simulink library "WECSim_Lib"  (R2014b)
settings: Solver=ode45  StartTime=0.0  StopTime=10.0  RelTol=1e-3
undefined symbols (not defined in the file): body, constraint, pto, simu, waves, X, Y, Z
libraries: nesl_utility x41, sm_lib x35
(part 2 of 2)

== system WECSim_Lib/PTOs/Translational PTO (Local Z) ==
  note: pto.loc
      | pto.c
      | pto.k
      | pto.name used in mask
  note: Constraints the motion to the desired DOF.
      | Applies PTO loads to the body based on PTO restoring and damping values.
      | Moves the connection points (B and F) from the free surface to the PTO location.
      | Calculates the PTO force and power.
      | Outputs forces, motions, and power.
  ForceAndPower : Subsystem
  Mux1 : Mux  Inputs=6
  PS-Simulink Converter{,1..3} (4 alike) : nesl_utility/PS-Simulink Converter  PhysicalDomain=network_engine_domain  SubClassName=ps_output  LeftPortType=input  RightPortType=output  PseudoPeriodic=off  Frequencies=[]  Unit=1  AffineConversion=off
  Rigid Transform : sm_lib/Frames and Transforms/Rigid Transform  TranslationMethod=Cartesian  TranslationLengthUnit=m  TranslationStandardAxis=+Z  TranslationStandardOffset=0  TranslationCartesianOffset=pto.loc  TranslationROffset=0  TranslationROffsetUnits=m  TranslationZOffset=0  TranslationZOffsetUnits=m  TranslationThetaOffset=0  TranslationThetaOffsetUnits=deg  RotationMethod=None  RotationAngleUnits=deg  RotationStandardAxis=+X  RotationAngle=90  RotationArbitraryAxis=[0 0 1]  FollAlignAxisA=+X  BaseAlignAxisA=+Y  FollAlignAxisB=+Y  BaseAlignAxisB=+Z  RotationMatrix=[1 0 0; 0 1 0; 0 0 1]  BlockFunction=simmechanics.library.frames_transforms.rigid_transform
  Rigid Transform1 : sm_lib/Frames and Transforms/Rigid Transform  TranslationMethod=Cartesian  TranslationLengthUnit=m  TranslationStandardAxis=+Z  TranslationStandardOffset=0  TranslationCartesianOffset=pto.loc  TranslationROffset=0  TranslationROffsetUnits=m  TranslationZOffset=0  TranslationZOffsetUnits=m  TranslationThetaOffset=0  TranslationThetaOffsetUnits=deg  RotationMethod=None  RotationAngleUnits=deg  RotationStandardAxis=+X  RotationAngle=90  RotationArbitraryAxis=[0 0 1]  FollAlignAxisA=+X  BaseAlignAxisA=+Y  FollAlignAxisB=+Y  BaseAlignAxisB=+Z  RotationMatrix=[1 0 0; 0 1 0; 0 0 1]  BlockFunction=simmechanics.library.frames_transforms.rigid_transform
  Translational PCC (Prismatic Joint) : sm_lib/Joints/Prismatic Joint  SenseConstraintForce=on  SenseConstraintForceX=off  SenseConstraintForceY=off  SenseConstraintForceZ=off  SenseConstraintTorque=on  SenseConstraintTorqueX=off  SenseConstraintTorqueY=off  SenseConstraintTorqueZ=off  SenseTotalForce=off  SenseTotalForceX=off  SenseTotalForceY=off  SenseTotalForceZ=off  SenseTotalTorque=off  SenseTotalTorqueX=off  SenseTotalTorqueY=off  SenseTotalTorqueZ=off  CompositeWrenchDir=BaseOnFollower  CompositeWrenchFrame=BaseFrame  EquilibriumPosition=0  EquilibriumPositionUnits=m  SpringStiffness=pto.k  SpringStiffnessUnits=N/m  DampingCoefficient=pto.c  DampingCoefficientUnits=N/(m/s)  TorqueActuationMode=NoTorque  MotionActuationMode=ComputedMotion  SensePosition=on  SenseVelocity=on  SenseAcceleration=off  SenseTorqueForce=off  PositionTargetValue=0  PositionTargetValueUnits=m  PositionTargetSpecify=off  PositionTargetPriority=High  VelocityTargetValue=0  VelocityTargetValueUnits=m/s  VelocityTargetSpecify=off  VelocityTargetPriority=High  BlockFunction=simmechanics.library.joints.prismatic_joint
  output : ToWorkspace  VariableName=PTO1_out  SaveFormat=Structure With Time  SampleTime=-1
  F : PMIOPort  Port=1  Side=Left
  B : PMIOPort  Port=2  Side=Right
  wires:
  PS-Simulink Converter1/1 -> Mux1/6, ForceAndPower/2(Vel)
  PS-Simulink Converter/1 -> Mux1/5, ForceAndPower/1(Pos)
  PS-Simulink Converter2/1 -> Mux1/3
  PS-Simulink Converter3/1 -> Mux1/4
  Mux1/1 -> output/1
  ForceAndPower/1(Force) -> Mux1/1
  ForceAndPower/2(Power) -> Mux1/2
  connections:
  Translational PCC (Prismatic Joint)/RConn3 -- PS-Simulink Converter1/LConn1
  Translational PCC (Prismatic Joint)/RConn2 -- PS-Simulink Converter/LConn1
  Translational PCC (Prismatic Joint)/RConn4 -- PS-Simulink Converter2/LConn1
  Translational PCC (Prismatic Joint)/RConn5 -- PS-Simulink Converter3/LConn1
  B/RConn1 -- Rigid Transform/LConn1
  Rigid Transform/RConn1 -- Translational PCC (Prismatic Joint)/LConn1
  Translational PCC (Prismatic Joint)/RConn1 -- Rigid Transform1/RConn1
  Rigid Transform1/LConn1 -- F/RConn1

== system WECSim_Lib/Body Elements/Rigid Body/Additional Linear Damping Force Calculation ==
  note: Calculates the additional linear damping force (if any)
      |
      | Additional Linear Damping Force = damping matrix (diagonal) * velocity vector = C * v
  Velocity : Inport
  Additional Linear Damping Matrix (diagonal) : Constant  Value=body.hydroForce.linearDamping
  Product1 : Product  Multiplication=Matrix(*)
  F_LinearDamping : Outport
  wires:
  Velocity/1 -> Product1/2  "v"
  Product1/1 -> F_LinearDamping/1  "F_LinearDamping"
  Additional Linear Damping Matrix (diagonal)/1 -> Product1/1  "C"

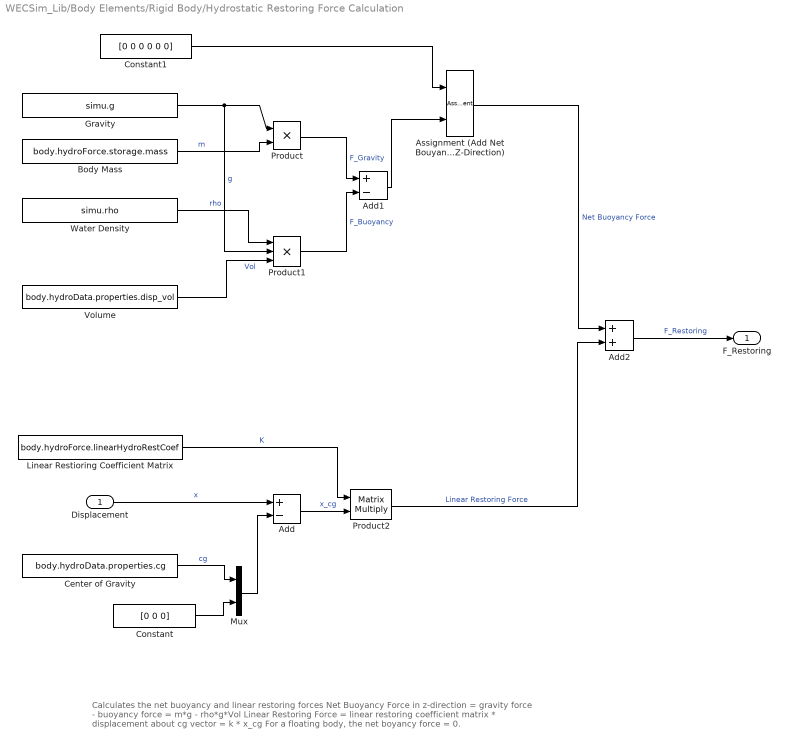
== system WECSim_Lib/Body Elements/Rigid Body/Hydrostatic Restoring Force Calculation ==
  note: Calculates the net buoyancy and linear restoring forces
      | 	Net Buoyancy Force in z-direction = gravity force - buoyancy force = m*g - rho*g*Vol
      | 	Linear Restoring Force = linear restoring coefficient matrix * displacement about cg vector = k * x_cg
      |
      | For a floating body, the net boyancy force = 0.
  Displacement : Inport
  Add : Sum  Inputs=+-
  Add1 : Sum  Inputs=+-
  Add2 : Sum
  Assignment (Add Net Bouyancy Force to Z-Direction) : Assignment  Indices=3
  Body Mass : Constant  Value=body.hydroForce.storage.mass
  Center of Gravity : Constant  Value=body.hydroData.properties.cg
  Constant : Constant  Value=[0 0 0]
  Constant1 : Constant  Value=[0 0 0 0 0 0]
  Gravity : Constant  Value=simu.g
  Linear Restioring Coefficient Matrix : Constant  Value=body.hydroForce.linearHydroRestCoef
  Mux : Mux  Inputs=2
  Product : Product
  Product1 : Product  Inputs=3
  Product2 : Product  Multiplication=Matrix(*)
  Volume : Constant  Value=body.hydroData.properties.disp_vol
  Water Density : Constant  Value=simu.rho
  F_Restoring : Outport
  wires:
  Add/1 -> Product2/2  "x_cg"
  Displacement/1 -> Add/1  "x"
  Mux/1 -> Add/2
  Center of Gravity/1 -> Mux/1  "cg"
  Constant/1 -> Mux/2
  Body Mass/1 -> Product/2  "m"
  Constant1/1 -> Assignment (Add Net Bouyancy Force to Z-Direction)/1
  Assignment (Add Net Bouyancy Force to Z-Direction)/1 -> Add2/1  "Net Buoyancy Force"
  Add2/1 -> F_Restoring/1  "F_Restoring"
  Volume/1 -> Product1/3  "Vol"
  Gravity/1 -> Product1/2, Product/1  "g"
  Water Density/1 -> Product1/1  "rho"
  Product/1 -> Add1/1  "F_Gravity"
  Product1/1 -> Add1/2  "F_Buoyancy"
  Add1/1 -> Assignment (Add Net Bouyancy Force to Z-Direction)/2
  Product2/1 -> Add2/2  "Linear Restoring Force"
  Linear Restioring Coefficient Matrix/1 -> Product2/1  "K"

== system WECSim_Lib/Body Elements/Rigid Body/Mooring Force Calculation (Map) ==
  note: Calculates the Mooring Force
      |
      | Mooring force = Kmooring matrix * displacement vector (relative to cg)
      | 	+ Cmooring matrix * velocity vector
      | 	- PreTension vector
      | F_Mooring = x_cg * Km  +  v * Cm  -  T
  Displacement : Inport
  Velocity : Inport  Port=2
  0 Disp for Rotation : Constant  Value=[0 0 0]
  Add : Sum  Inputs=+-
  Center of Gravity : Constant  Value=body.hydroData.properties.cg
  Center of Gravity2 : Constant  Value=body.mooring.c
  Mooring K Matrix : Constant  Value=body.mooring.k
  Mooring Pre-Tension : Constant  Value=body.mooring.preTension
  Mux : Mux  Inputs=2
  Product : Product  Multiplication=Matrix(*)
  Product1 : Product  Multiplication=Matrix(*)
  sum : Sum  Inputs=++-
  F_Mooring : Outport
  wires:
  Product/1 -> sum/1  "Km*x_cg"
  Product1/1 -> sum/2  "Cm*v"
  sum/1 -> F_Mooring/1  "F_Mooring"
  Mooring Pre-Tension/1 -> sum/3  "T"
  Add/1 -> Product/2  "x_cg"
  Mux/1 -> Add/2
  Displacement/1 -> Add/1  "x"
  Center of Gravity/1 -> Mux/1  "cg"
  Mooring K Matrix/1 -> Product/1  "Km"
  Velocity/1 -> Product1/2  "v"
  Center of Gravity2/1 -> Product1/1  "Cm"
  0 Disp for Rotation/1 -> Mux/2

== system WECSim_Lib/Body Elements/Rigid Body/Structure ==
  note: body.mass
      | body.momOfInertia
      | body.geometryFile (set through Rigid Body mask)
      | body.hydroData.properties.cg
      | body.initDisp.initAngularDispAxis
      | body.initDisp.initAngularDispAngle
      | body.initDisp.initLinDisp
  note: SimMechanics Model
      |
      | Body: Consists of body properties (inertia and vizualisation) defined at the CG, and a connection point at (0,0,0), the free surface.
      |
      | Forces::  Total forces calculated by WEC-Sim are applied at the Body CG. Other forces (constraints and PTOs) can be applied outside of this block, though the connection point.
      |
      | Motion Sensor: Measures the displacement, velocity, and acceleration of the Body CG relative to the world frame.
  Total Force : Inport
  Body Properties : sm_lib/Body Elements/Solid  InertiaType=Custom  Mass=body.mass  MassUnits=kg  CenterOfMass=[0 0 0]  CenterOfMassUnits=m  MomentsOfInertia=body.momOfInertia  MomentsOfInertiaUnits=kg*m^2  ProductsOfInertia=[0 0 0]  ProductsOfInertiaUnits=kg*m^2  DensityBased=on  Density=1000  DensityUnits=kg/(m^3)  GraphicType=FromGeometry  MarkerShape=Sphere  MarkerSize=10  MarkerSizeUnits=m  GraphicVisPropType=SimpleVisualProperties  GraphicDiffuseColor=[1 1 0]  GraphicSpecularColor=[0.5 0.5 0.5 1.0]  GraphicAmbientColor=[0.15 0.15 0.15 1.0]  GraphicEmissiveColor=[0.0 0.0 0.0 1.0]  GraphicShininess=75  GraphicOpacity=1  GeometryShape=FromFile  RectangleSize=[1 1]  RectangleSizeUnits=m  BrickDimensions=[1 1 1]  BrickDimensionUnits=m  CylinderRadius=1  CylinderRadiusUnits=m  CylinderLength=1  CylinderLengthUnits=m  SphereRadius=1  SphereRadiusUnits=m  EllipsoidRadii=[1 1 1]  EllipsoidRadiiUnits=m  ExtrusionCrossSection=[1 1; -1 1; -1 -1; 1 -1]  ExtrusionCrossSectionUnits=m  ExtrusionLength=1  ExtrusionLengthUnits=m  PolygonNumSides=3  PolygonOuterRadius=1  PolygonOuterRadiusUnits=m  ExtGeomFileType=STL  ExtGeomFileName=geometry/flap.stl  ExtGeomFileUnits=m  RevolutionCrossSection=[1 1; 1 -1; 2 -1; 2 1]  RevolutionCrossSectionUnits=m  RevolutionExtent=Full  RevolutionAngle=180  RevolutionAngleUnits=deg  BlockFunction=simmechanics.library.body_elements.solid
  External Force and Torque : sm_lib/Forces and Torques/External Force and Torque  ForceResolutionFrame=AttachedFrame  EnableForceX=off  EnableForceY=off  EnableForceZ=off  EnableForce=on  TorqueResolutionFrame=AttachedFrame  EnableTorqueX=off  EnableTorqueY=off  EnableTorqueZ=off  EnableTorque=on  BlockFunction=simmechanics.library.forces_torques.external_force_torque
  Motion Sensor : Subsystem
  Rigid Transform (Setup CG) : sm_lib/Frames and Transforms/Rigid Transform  TranslationMethod=Cartesian  TranslationLengthUnit=m  TranslationStandardAxis=+Z  TranslationStandardOffset=0  TranslationCartesianOffset=body.hydroData.properties.cg  TranslationROffset=0  TranslationROffsetUnits=m  TranslationZOffset=0  TranslationZOffsetUnits=m  TranslationThetaOffset=0  TranslationThetaOffsetUnits=deg  RotationMethod=None  RotationAngleUnits=rad  RotationStandardAxis=+Y  RotationAngle=0.05  RotationArbitraryAxis=[0.57735026918962584 0.57735026918962584 0.57735026918962584]  FollAlignAxisA=+X  BaseAlignAxisA=+Y  FollAlignAxisB=+Y  BaseAlignAxisB=+Z  RotationMatrix=[1 0 0; 0 1 0; 0 0 1]  BlockFunction=simmechanics.library.frames_transforms.rigid_transform
  Rigid Transform (Setup Initial Disp) : sm_lib/Frames and Transforms/Rigid Transform  TranslationMethod=Cartesian  TranslationLengthUnit=m  TranslationStandardAxis=+Z  TranslationStandardOffset=0  TranslationCartesianOffset=body.initDisp.initLinDisp  TranslationROffset=0  TranslationROffsetUnits=m  TranslationZOffset=0  TranslationZOffsetUnits=m  TranslationThetaOffset=0  TranslationThetaOffsetUnits=deg  RotationMethod=ArbitraryAxis  RotationAngleUnits=rad  RotationStandardAxis=+Y  RotationAngle=body.initDisp.initAngularDispAngle  RotationArbitraryAxis=body.initDisp.initAngularDispAxis  FollAlignAxisA=+X  BaseAlignAxisA=+Y  FollAlignAxisB=+Y  BaseAlignAxisB=+Z  RotationMatrix=[1 0 0; 0 1 0; 0 0 1]  BlockFunction=simmechanics.library.frames_transforms.rigid_transform
  Selector : Selector  InputPortWidth=6  Indices=[1:3]
  Selector1 : Selector  InputPortWidth=6  Indices=[4:6]
  Simulink-PS Converter1 : nesl_utility/Simulink-PS Converter  PhysicalDomain=network_engine_domain  SubClassName=ps_input  LeftPortType=input  RightPortType=output  PseudoPeriodic=off  Frequencies=[]  NoiseDistribution=none  NoiseParameters=[]  Unit=1  AffineConversion=off  InputFiltering=off  SimscapeFilterOrder=1  InputFilterTimeConstant=0.001  UdotUserProvided=1
  Simulink-PS Converter2 : nesl_utility/Simulink-PS Converter  PhysicalDomain=network_engine_domain  SubClassName=ps_input  LeftPortType=input  RightPortType=output  PseudoPeriodic=off  Frequencies=[]  NoiseDistribution=none  NoiseParameters=[]  Unit=1  AffineConversion=off  InputFiltering=off  SimscapeFilterOrder=1  InputFilterTimeConstant=0.001  UdotUserProvided=1
  World Frame : sm_lib/Frames and Transforms/World Frame  BlockFunction=simmechanics.library.frames_transforms.world_frame
  Conn Free Surface : PMIOPort  Port=1  Side=Right
  Response : Outport
  wires:
  Total Force/1 -> Selector1/1, Selector/1
  Selector/1 -> Simulink-PS Converter1/1
  Selector1/1 -> Simulink-PS Converter2/1
  Motion Sensor/1(Response) -> Response/1
  connections:
  External Force and Torque/LConn1 -- Simulink-PS Converter1/RConn1
  External Force and Torque/LConn2 -- Simulink-PS Converter2/RConn1
  Rigid Transform (Setup Initial Disp)/RConn1 -- Body Properties/RConn1 -- External Force and Torque/RConn1 -- Motion Sensor/RConn1
  Conn Free Surface/RConn1 -- Rigid Transform (Setup CG)/LConn1
  Rigid Transform (Setup Initial Disp)/LConn1 -- Rigid Transform (Setup CG)/RConn1
  World Frame/RConn1 -- Motion Sensor/LConn1

== system WECSim_Lib/Body Elements/Rigid Body/Viscous Damping Force Calculation ==
  note: Calculates Viscous Drag (Quadratic) Force
      |
      | Viscous Drag Force = 1/2 * drag coefficient * water density * characteristic area * velocity squared (signed) = 0.5 * cd * rho *A * v * |v|
  Velocity : Inport
  Abs : Abs
  Product : Product
  Product1 : Product  Multiplication=Matrix(*)
  "Viscous Damping Matrix (diagonal) " : Constant  Value=body.hydroForce.visDrag
  F_Viscous : Outport
  wires:
  Velocity/1 -> Product/1, Abs/1
  Abs/1 -> Product/2
  Product1/1 -> F_Viscous/1  "F_Viscous"
  "Viscous Damping Matrix (diagonal) "/1 -> Product1/1  "0.5 * cd * rho *A"
  Product/1 -> Product1/2  "v * |v|"

== system WECSim_Lib/Body Elements/Rigid Body/Wave Diffraction and Excitation Force Calculation ==
  note: Calculates the excitation force, F_Excitation, given by
      | F_Excitation = R * F_wave.
      |
      | There are two cases for Calculating the Ramp function, R:
      |    1. simulation Time is less than Ramp Time: Apply ramp function
      |    2. Simulation time is larger than Ramp Time: Do not apply ramp function (R=1)
      |
      | Similarly there are two cases for the wave force, F_wave: Regular and Irregular waves.
      |
      | Notes:
      | Output dimension set to '6' in output port to eliminate singleton dimension.
  Time : Inport
  If : If  IfExpression=u1 < 20
  If1 : If  NumInputs=2  IfExpression=u1 < u2
  Iregular Wave Excitation Force : Subsystem  TreatAsAtomicUnit=on
  Merge : Merge
  Merge1 : Merge
  No Ramp Function : Subsystem  TreatAsAtomicUnit=on
  Product : Product
  Ramp Function : Subsystem  TreatAsAtomicUnit=on
  Ramp Function Time : Constant  Value=simu.rampT
  Regular Wave Excitation Force : Subsystem  TreatAsAtomicUnit=on
  Wave Type : Constant  Value=waves.typeNum
  F_Excitation : Outport  PortDimensions=6
  wires:
  No Ramp Function/1(R) -> Merge1/2
  Ramp Function/1(R) -> Merge1/1
  If1/1 -> Ramp Function/Action
  If1/2 -> No Ramp Function/Action
  Ramp Function Time/1 -> If1/2
  Iregular Wave Excitation Force/1(F_wave) -> Merge/2
  Regular Wave Excitation Force/1(F_wave) -> Merge/1
  If/2 -> Iregular Wave Excitation Force/Action
  If/1 -> Regular Wave Excitation Force/Action
  Wave Type/1 -> If/1
  Merge/1 -> Product/2  "F_wave"
  Merge1/1 -> Product/1  "R"
  Product/1 -> F_Excitation/1  "F_Excitation"
  Time/1 -> Ramp Function/1(Time), If1/1, Iregular Wave Excitation Force/1(Time), Regular Wave Excitation Force/1(Time)

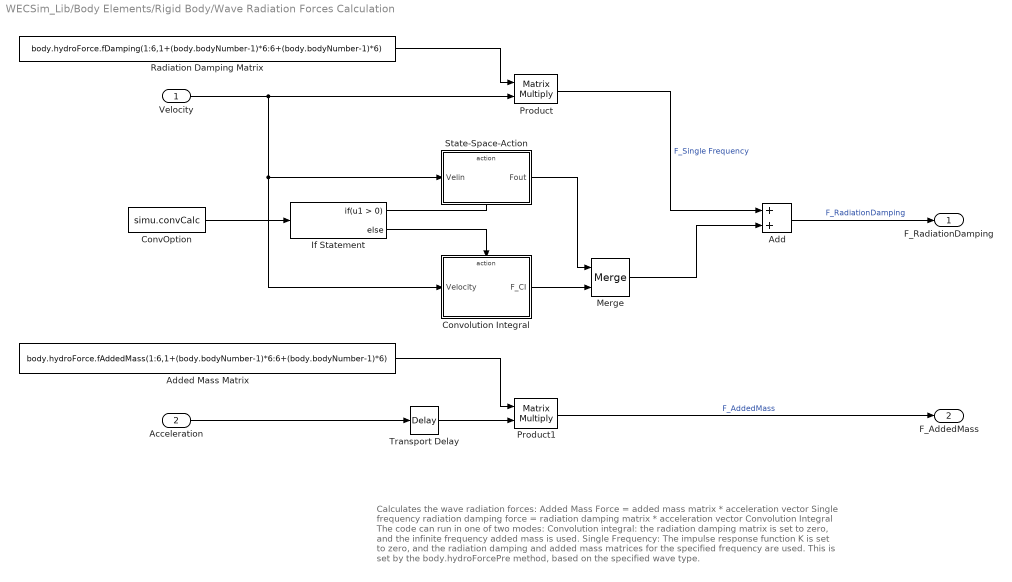
== system WECSim_Lib/Body Elements/Rigid Body/Wave Radiation Forces Calculation ==
  note: Calculates the wave radiation forces:
      | 	Added Mass Force = added mass matrix * acceleration vector
      | 	Single frequency radiation damping force = radiation damping matrix * acceleration vector
      | 	Convolution Integral
      |
      | The code can run in one of two modes:
      | 	Convolution integral: the radiation damping matrix is set to zero, and the infinite frequency added mass is used.
      | 	Single Frequency: The impulse response function K is set to zero, and the radiation damping and added mass matrices for the specified frequency are used.
      |
      | This is set by the body.hydroForcePre method, based on the specified wave type.
  Velocity : Inport
  Acceleration : Inport  Port=2
  Add : Sum
  Added Mass Matrix : Constant  Value=body.hydroForce.fAddedMass(1:6,1+(body.bodyNumber-1)*6:6+(body.bodyNumber-1)*6)
  ConvOption : Constant  Value=simu.convCalc
  Convolution Integral : Subsystem
  If Statement : If
  Merge : Merge
  Product : Product  Multiplication=Matrix(*)
  Product1 : Product  Multiplication=Matrix(*)
  Radiation Damping Matrix : Constant  Value=body.hydroForce.fDamping(1:6,1+(body.bodyNumber-1)*6:6+(body.bodyNumber-1)*6)
  State-Space-Action : Subsystem  TreatAsAtomicUnit=on
  Transport Delay : TransportDelay  DelayTime=10e-8
  F_RadiationDamping : Outport
  F_AddedMass : Outport  Port=2
  wires:
  Acceleration/1 -> Transport Delay/1
  Transport Delay/1 -> Product1/2
  Add/1 -> F_RadiationDamping/1  "F_RadiationDamping"
  Velocity/1 -> Convolution Integral/1(Velocity), State-Space-Action/1(Velin), Product/2
  Product/1 -> Add/1  "F_Single Frequency"
  Product1/1 -> F_AddedMass/1  "F_AddedMass"
  Radiation Damping Matrix/1 -> Product/1
  Added Mass Matrix/1 -> Product1/1
  If Statement/2 -> Convolution Integral/Action
  If Statement/1 -> State-Space-Action/Action
  State-Space-Action/1(Fout) -> Merge/1
  Convolution Integral/1(F_CI) -> Merge/2
  ConvOption/1 -> If Statement/1
  Merge/1 -> Add/2

== system WECSim_Lib/PTOs/Rotational PTO (Local RY)/ForceAndPower ==
  note: Calculate PTO force and power.
      |
      | F_pto  = k*x + c*v,
      | where F_pto is the force the PTO applies to the body (at the PTO location), x and v are the joint position and velocity.
      |
      | The power extracted is
      | P = c * v^2
  Pos : Inport
  Vel : Inport  Port=2
  Add : Sum
  Math Function : Math  Operator=square  SaturateOnIntegerOverflow=on
  PCC Damping Coefficient : Constant  Value=pto.c
  PCC Stiffness Coefficient : Constant  Value=pto.k
  Product : Product  Inputs=**
  Product1 : Product  Inputs=**
  Product2 : Product  Inputs=**
  Force/Torque : Outport
  Power : Outport  Port=2
  wires:
  PCC Damping Coefficient/1 -> Product2/1, Product1/1
  Product2/1 -> Power/1
  Vel/1 -> Math Function/1, Product1/2
  PCC Stiffness Coefficient/1 -> Product/2
  Pos/1 -> Product/1
  Add/1 -> Force/Torque/1
  Math Function/1 -> Product2/2
  Product/1 -> Add/1
  Product1/1 -> Add/2

== system WECSim_Lib/PTOs/Translational PTO (Local X)/ForceAndPower ==
  note: Calculate PTO force and power.
      |
      | F_pto  = k*x + c*v,
      | where F_pto is the force the PTO applies to the body (at the PTO location), x and v are the joint position and velocity.
      |
      | The power extracted is
      | P = c * v^2
  Pos : Inport
  Vel : Inport  Port=2
  Add : Sum
  Math Function : Math  Operator=square  SaturateOnIntegerOverflow=on
  PCC Damping Coefficient : Constant  Value=pto.c
  PCC Stiffness Coefficient : Constant  Value=pto.k
  Product : Product  Inputs=**
  Product1 : Product  Inputs=**
  Product2 : Product  Inputs=**
  Force : Outport
  Power : Outport  Port=2
  wires:
  PCC Damping Coefficient/1 -> Product1/1, Product2/1
  Product2/1 -> Power/1
  Vel/1 -> Product1/2, Math Function/1
  PCC Stiffness Coefficient/1 -> Product/2
  Pos/1 -> Product/1
  Add/1 -> Force/1
  Math Function/1 -> Product2/2
  Product/1 -> Add/1
  Product1/1 -> Add/2

== system WECSim_Lib/PTOs/Translational PTO (Local Z)/ForceAndPower ==
  note: Calculate PTO force and power.
      |
      | F_pto  = k*x + c*v,
      | where F_pto is the force the PTO applies to the body (at the PTO location), x and v are the joint position and velocity.
      |
      | The power extracted is
      | P = c * v^2
  Pos : Inport
  Vel : Inport  Port=2
  Add : Sum
  Math Function : Math  Operator=square  SaturateOnIntegerOverflow=on
  PCC Damping Coefficient : Constant  Value=pto.c
  PCC Stiffness Coefficient : Constant  Value=pto.k
  Product : Product  Inputs=**
  Product1 : Product  Inputs=**
  Product2 : Product  Inputs=**
  Force : Outport
  Power : Outport  Port=2
  wires:
  PCC Damping Coefficient/1 -> Product2/1, Product1/1
  Product2/1 -> Power/1
  Vel/1 -> Math Function/1, Product1/2
  PCC Stiffness Coefficient/1 -> Product/2
  Pos/1 -> Product/1
  Add/1 -> Force/1
  Math Function/1 -> Product2/2
  Product/1 -> Add/1
  Product1/1 -> Add/2

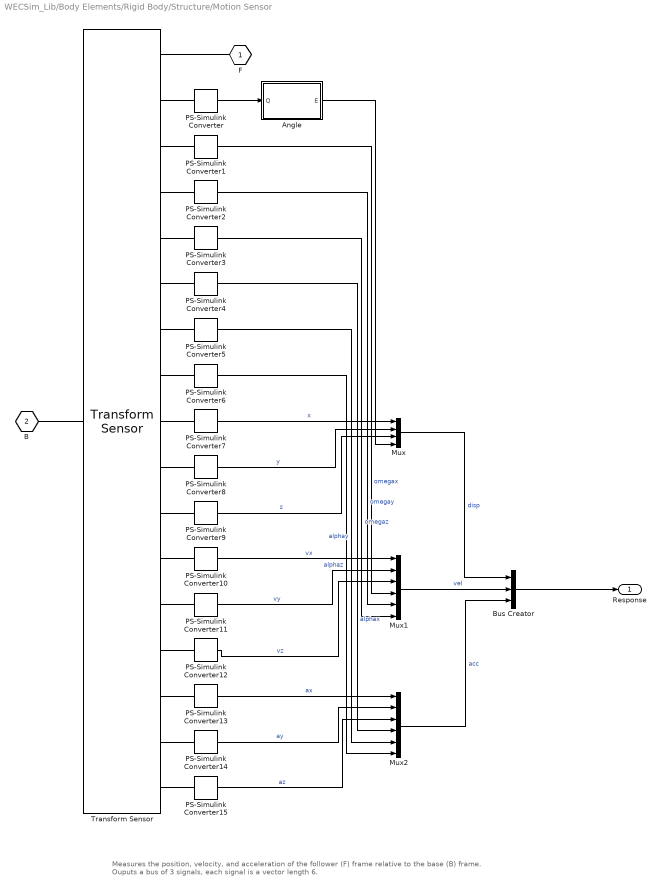
== system WECSim_Lib/Body Elements/Rigid Body/Structure/Motion Sensor ==
  note: Measures the position, velocity, and acceleration of the follower (F) frame relative to the base (B) frame.
      | Ouputs a bus of 3 signals, each signal is a vector length 6.
  Angle : MATLAB Function  TreatAsAtomicUnit=on
  Bus Creator : BusCreator  Inputs=3
  Mux : Mux
  Mux1 : Mux  Inputs=6
  Mux2 : Mux  Inputs=6
  PS-Simulink Converter{,1..15} (16 alike) : nesl_utility/PS-Simulink Converter  PhysicalDomain=network_engine_domain  SubClassName=ps_output  LeftPortType=input  RightPortType=output  PseudoPeriodic=off  Frequencies=[]  Unit=1  AffineConversion=off
  Transform Sensor : sm_lib/Frames and Transforms/Transform Sensor  MeasurementFrame=World  SenseAngle=off  SenseAxis=off  SenseAngle1=off  SenseAngle2=off  SenseAngle3=off  SenseQ=on  SenseR=off  SenseOmegaX=on  SenseOmegaY=on  SenseOmegaZ=on  SenseOmega1=off  SenseOmega2=off  SenseOmega3=off  SenseQDot=off  SenseRDot=off  SenseAlphaX=on  SenseAlphaY=on  SenseAlphaZ=on  SenseAlpha1=off  SenseAlpha2=off  SenseAlpha3=off  SenseQDDot=off  SenseRDDot=off  SenseX=on  SenseY=on  SenseZ=on  SenseRad=off  SenseAzim=off  SenseDist=off  SenseInc=off  SenseXDot=on  SenseYDot=on  SenseZDot=on  SenseRadDot=off  SenseAzimDot=off  SenseDistDot=off  SenseIncDot=off  SenseXDDot=on  SenseYDDot=on  SenseZDDot=on  SenseRadDDot=off  SenseAzimDDot=off  SenseDistDDot=off  SenseIncDDot=off  BlockFunction=simmechanics.library.frames_transforms.transform_sensor
  F : PMIOPort  Port=1  Side=Right
  B : PMIOPort  Port=2  Side=Left
  Response : Outport
  wires:
  PS-Simulink Converter/1 -> Angle/1(Q)
  PS-Simulink Converter4/1 -> Mux2/4  "alphax"
  PS-Simulink Converter10/1 -> Mux1/1  "vx"
  PS-Simulink Converter12/1 -> Mux1/3  "vz"
  PS-Simulink Converter13/1 -> Mux2/1  "ax"
  PS-Simulink Converter14/1 -> Mux2/2  "ay"
  Mux/1 -> Bus Creator/1  "disp"
  Mux1/1 -> Bus Creator/2  "vel"
  Mux2/1 -> Bus Creator/3  "acc"
  Angle/1(E) -> Mux/4
  PS-Simulink Converter7/1 -> Mux/1  "x"
  PS-Simulink Converter8/1 -> Mux/2  "y"
  PS-Simulink Converter9/1 -> Mux/3  "z"
  PS-Simulink Converter5/1 -> Mux2/5  "alphay"
  PS-Simulink Converter6/1 -> Mux2/6  "alphaz"
  PS-Simulink Converter1/1 -> Mux1/4  "omegax"
  PS-Simulink Converter2/1 -> Mux1/5  "omegay"
  PS-Simulink Converter11/1 -> Mux1/2  "vy"
  PS-Simulink Converter3/1 -> Mux1/6  "omegaz"
  PS-Simulink Converter15/1 -> Mux2/3  "az"
  Bus Creator/1 -> Response/1
  connections:
  Transform Sensor/RConn1 -- F/RConn1
  B/RConn1 -- Transform Sensor/LConn1
  Transform Sensor/RConn2 -- PS-Simulink Converter/LConn1
  PS-Simulink Converter15/LConn1 -- Transform Sensor/RConn17
  PS-Simulink Converter14/LConn1 -- Transform Sensor/RConn16
  PS-Simulink Converter13/LConn1 -- Transform Sensor/RConn15
  PS-Simulink Converter12/LConn1 -- Transform Sensor/RConn14
  PS-Simulink Converter11/LConn1 -- Transform Sensor/RConn13
  PS-Simulink Converter10/LConn1 -- Transform Sensor/RConn12
  PS-Simulink Converter9/LConn1 -- Transform Sensor/RConn11
  PS-Simulink Converter8/LConn1 -- Transform Sensor/RConn10
  PS-Simulink Converter7/LConn1 -- Transform Sensor/RConn9
  PS-Simulink Converter4/LConn1 -- Transform Sensor/RConn6
  PS-Simulink Converter5/LConn1 -- Transform Sensor/RConn7
  PS-Simulink Converter6/LConn1 -- Transform Sensor/RConn8
  PS-Simulink Converter1/LConn1 -- Transform Sensor/RConn3
  PS-Simulink Converter2/LConn1 -- Transform Sensor/RConn4
  PS-Simulink Converter3/LConn1 -- Transform Sensor/RConn5

== system WECSim_Lib/Body Elements/Rigid Body/Wave Diffraction and Excitation Force Calculation/Iregular Wave Excitation Force ==
  note: Calculates the wave force, F_wave, for the case of Irregular Waves.
      |
      | F_wave = sum( F_wave(i))
      |
      | where i = each frequency bin.
  Time : Inport
  Action Port : ActionPort
  For Each Subsystem : Subsystem  TreatAsAtomicUnit=on
  Imaginary Part of Wave Excitation : Constant  Value=body.hydroForce.fExt.im  VectorParams1D=off
  Random Phase : Constant  Value=waves.phaseRand  VectorParams1D=off
  Real Part of Wave Excitation : Constant  Value=body.hydroForce.fExt.re  VectorParams1D=off
  Sum of Elements : Sum  Inputs=+  CollapseMode=Specified dimension
  Wave Frequency : Constant  Value=waves.w  VectorParams1D=off
  Wave Spectrum : Constant  Value=waves.A  VectorParams1D=off
  F_wave : Outport
  wires:
  Random Phase/1 -> For Each Subsystem/5(Random Phase)
  Sum of Elements/1 -> F_wave/1
  For Each Subsystem/1(F_wave(i)) -> Sum of Elements/1
  Wave Frequency/1 -> For Each Subsystem/2(Wave Frequency)
  Imaginary Part of Wave Excitation/1 -> For Each Subsystem/4(Imaginary Part of Wave Excitation)
  Real Part of Wave Excitation/1 -> For Each Subsystem/3(Real Part of Wave Excitation)
  Wave Spectrum/1 -> For Each Subsystem/1(Wave Spectrum)
  Time/1 -> For Each Subsystem/6(Time)

== system WECSim_Lib/Body Elements/Rigid Body/Wave Diffraction and Excitation Force Calculation/No Ramp Function ==
  note: No ramp function applied.
      | R = 1
      |
      | Note:
      | Output port initial value also set to 1,
  Action Port : ActionPort
  Constant : Constant
  R : Outport  InitialOutput=1
  wires:
  Constant/1 -> R/1

== system WECSim_Lib/Body Elements/Rigid Body/Wave Diffraction and Excitation Force Calculation/Ramp Function ==
  note: Calculates the ramp function, R, given by
      |
      | R = (1 / 2)  * (1 + sin( (pi / t_ramp) * t  +  ((3 / 2) * pi) ) ).
  Time : Inport
  Action Port : ActionPort
  Add : Sum
  Add1 : Sum
  Constant : Constant  Value=1/2
  Constant1 : Constant
  Constant2 : Constant  Value=3*pi/2
  Constant3 : Constant  Value=pi
  Divide : Product  Inputs=*/
  Product : Product
  Product1 : Product
  Ramp Time : Constant  Value=simu.rampT
  Sine Wave Function : Sin  TimeSource=Use external signal  SampleTime=0
  R : Outport
  wires:
  Add/1 -> Product/1
  Sine Wave Function/1 -> Add/2
  Constant1/1 -> Add/1
  Constant/1 -> Product/2
  Product/1 -> R/1
  Time/1 -> Product1/1  "t"
  Ramp Time/1 -> Divide/2  "t_ramp"
  Constant2/1 -> Add1/2  "phase"
  Add1/1 -> Sine Wave Function/1
  Product1/1 -> Add1/1
  Constant3/1 -> Divide/1
  Divide/1 -> Product1/2  "frequency"

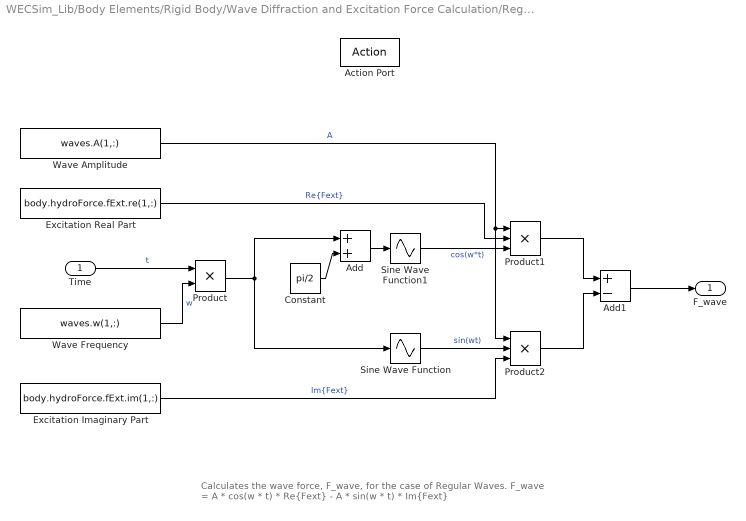
== system WECSim_Lib/Body Elements/Rigid Body/Wave Diffraction and Excitation Force Calculation/Regular Wave Excitation Force ==
  note: Calculates the wave force, F_wave, for the case of Regular Waves.
      |
      | F_wave =   A * cos(w * t) * Re{Fext}
      |                -  A * sin(w * t) * Im{Fext}
  Time : Inport
  Action Port : ActionPort
  Add : Sum
  Add1 : Sum  Inputs=+-
  Constant : Constant  Value=pi/2
  Excitation Imaginary Part : Constant  Value=body.hydroForce.fExt.im(1,:)  VectorParams1D=off
  Excitation Real Part : Constant  Value=body.hydroForce.fExt.re(1,:)  VectorParams1D=off
  Product : Product
  Product1 : Product  Inputs=3
  Product2 : Product  Inputs=3
  Sine Wave Function : Sin  TimeSource=Use external signal  SampleTime=0
  Sine Wave Function1 : Sin  TimeSource=Use external signal  SampleTime=0
  Wave Amplitude : Constant  Value=waves.A(1,:)
  Wave Frequency : Constant  Value=waves.w(1,:)
  F_wave : Outport
  wires:
  Time/1 -> Product/1  "t"
  Wave Frequency/1 -> Product/2  "w"
  Product/1 -> Sine Wave Function/1, Add/1
  Sine Wave Function1/1 -> Product1/3  "cos(w*t)"
  Sine Wave Function/1 -> Product2/2  "sin(wt)"
  Excitation Imaginary Part/1 -> Product2/3  "Im{Fext}"
  Excitation Real Part/1 -> Product1/2  "Re{Fext}"
  Product1/1 -> Add1/1
  Product2/1 -> Add1/2
  Add1/1 -> F_wave/1
  Wave Amplitude/1 -> Product2/1, Product1/1  "A"
  Add/1 -> Sine Wave Function1/1
  Constant/1 -> Add/2

== system WECSim_Lib/Body Elements/Rigid Body/Wave Radiation Forces Calculation/Convolution Integral ==
  Velocity : Inport
  Action Port : ActionPort
  Fluid Memory1 : MATLAB Function  TreatAsAtomicUnit=on
  Impulse Response Function K1 : Constant  Value=body.hydroForce.irkb(:,1:6,1+(body.bodyNumber-1)*6:6+(body.bodyNumber-1)*6)
  Time (relative to the current time step)1 : Constant  Value=simu.CTTime
  Wave Type1 : Constant  Value=waves.typeNum
  F_CI : Outport
  wires:
  Wave Type1/1 -> Fluid Memory1/1(check)
  Time (relative to the current time step)1/1 -> Fluid Memory1/4(CTTime)
  Impulse Response Function K1/1 -> Fluid Memory1/3(IRKB)
  Velocity/1 -> Fluid Memory1/2(v)
  Fluid Memory1/1(F_FM) -> F_CI/1  "F_Convolution Integral"

== system WECSim_Lib/Body Elements/Rigid Body/Wave Radiation Forces Calculation/State-Space-Action ==
  Velin : Inport
  Action Port : ActionPort
  State-Space : StateSpace  A=body.hydroForce.ssRadf.A  B=body.hydroForce.ssRadf.B  C=body.hydroForce.ssRadf.C  D=body.hydroForce.ssRadf.D  X0=0
  Fout : Outport
  wires:
  Velin/1 -> State-Space/1
  State-Space/1 -> Fout/1

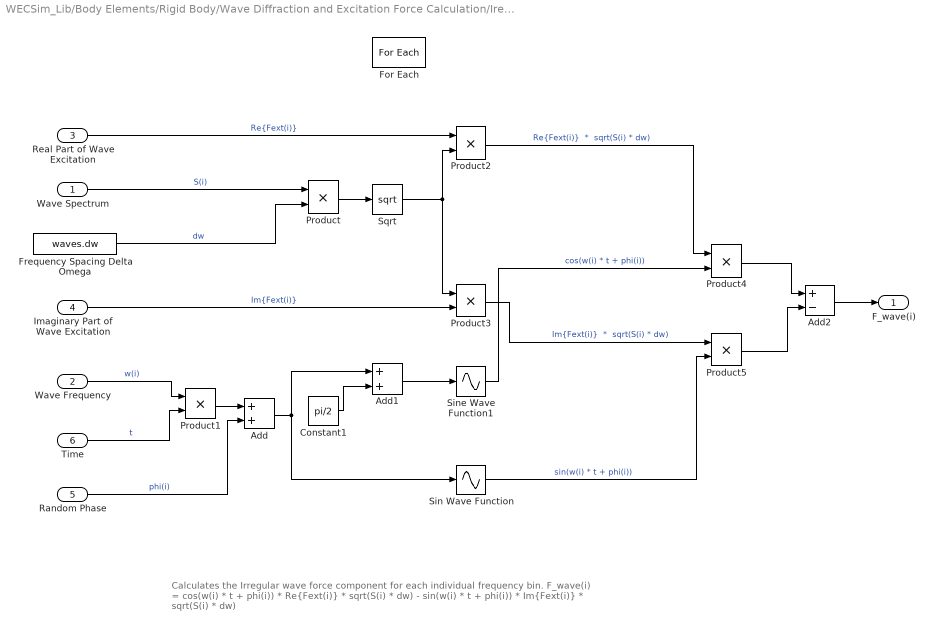
== system WECSim_Lib/Body Elements/Rigid Body/Wave Diffraction and Excitation Force Calculation/Iregular Wave Excitation Force/For Each Subsystem ==
  note: Calculates the Irregular wave force component for each individual frequency bin.
      |
      | F_wave(i) =  cos(w(i) * t + phi(i))  *  Re{Fext(i)}  *  sqrt(S(i) * dw)
      |                    - sin(w(i) * t + phi(i))  *  Im{Fext(i)}  *  sqrt(S(i) * dw)
  Wave Spectrum : Inport  Partition=on  PartitionDimension=1  PartitionWidth=1
  Wave Frequency : Inport  Port=2  Partition=on  PartitionDimension=1  PartitionWidth=1
  Real Part of Wave Excitation : Inport  Port=3  Partition=on  PartitionDimension=1  PartitionWidth=1
  Imaginary Part of Wave Excitation : Inport  Port=4  Partition=on  PartitionDimension=1  PartitionWidth=1
  Random Phase : Inport  Port=5  Partition=on  PartitionDimension=1  PartitionWidth=1
  Time : Inport  Port=6  Partition=off
  Add : Sum
  Add1 : Sum
  Add2 : Sum  Inputs=+-
  Constant1 : Constant  Value=pi/2
  For Each : ForEach  DisableCoverage=on  IndexMode=One-based
  Frequency Spacing Delta Omega : Constant  Value=waves.dw  VectorParams1D=off
  Product{,1..5} (6 alike) : Product  Inputs=**
  Sin Wave Function : Sin  TimeSource=Use external signal  SampleTime=0
  Sine Wave Function1 : Sin  TimeSource=Use external signal  SampleTime=0
  Sqrt : Sqrt  SaturateOnIntegerOverflow=on
  F_wave(i) : Outport  ConcatenationDimension=1
  wires:
  Add/1 -> Sin Wave Function/1, Add1/1
  Random Phase/1 -> Add/2  "phi(i)"
  Product1/1 -> Add/1
  Sqrt/1 -> Product3/1, Product2/2
  Product/1 -> Sqrt/1
  Frequency Spacing Delta Omega/1 -> Product/2  "dw"
  Wave Spectrum/1 -> Product/1  "S(i)"
  Time/1 -> Product1/2  "t"
  Add2/1 -> F_wave(i)/1
  Wave Frequency/1 -> Product1/1  "w(i)"
  Real Part of Wave Excitation/1 -> Product2/1  "Re{Fext(i)}"
  Imaginary Part of Wave Excitation/1 -> Product3/2  "Im{Fext(i)}"
  Product5/1 -> Add2/2
  Product4/1 -> Add2/1
  Product2/1 -> Product4/1  "Re{Fext(i)}  *  sqrt(S(i) * dw)"
  Product3/1 -> Product5/1  "Im{Fext(i)}  *  sqrt(S(i) * dw)"
  Sine Wave Function1/1 -> Product4/2  "cos(w(i) * t + phi(i))"
  Sin Wave Function/1 -> Product5/2  "sin(w(i) * t + phi(i))"
  Add1/1 -> Sine Wave Function1/1
  Constant1/1 -> Add1/2

== matlab function WECSim_Lib/Body Elements/Rigid Body/Wave Radiation Forces Calculation/Convolution Integral/Fluid Memory1 ==
  data: check input; v input; F_FM output; IRKB input; CTTime input
function F_FM = ConvolutionalIntegral(check,v,IRKB,CTTime)

%define persistent variables
persistent velocity;
persistent kkk
len = length(CTTime);

if check==10
    tmpT = zeros(6,1);
else
    if isempty(velocity)
       velocity = zeros(6,len);
       kkk=0;
    else
       kkk=kkk+1;         
       int2=abs(kkk-floor(kkk/5)*5-1);
       if int2<0.00000001
          velocity(:,2:end) = velocity(:,1:end-1);
       end
       velocity(:,1) = v(:);
    end 
    
	%integrate
    tmpT = zeros(6,1);
    for kd=1:6
        tmpV = zeros(len,1);
        for kk=1:6
            tmpY=IRKB(:,kd,kk).*velocity(kk,:)';
            tmpV = tmpV + tmpY;
        end
        tmpT(kd) = trapz(CTTime,tmpV);
    end
end
F_FM=tmpT;
end

== matlab function WECSim_Lib/Body Elements/Rigid Body/Structure/Motion Sensor/Angle ==
  data: Q input; E output
function E  = EulerAngle(Q)
%#codegen
E=zeros(3,1);
E(1) = atan2( (2*(Q(1)*Q(2)+Q(3)*Q(4))), (1-2* (Q(2)^2+Q(3)^2) ) );
E(2) = asin( 2* (Q(1)*Q(3) - Q(4)*Q(2)));
E(3) = atan2( (2*(Q(1)*Q(4)+Q(2)*Q(3))), (1-2* (Q(3)^2+Q(4)^2) ) );
